simulink model "Frequency_Shift_Keying"  (R2023b)
settings: Solver=VariableStepAuto  StartTime=0.0  StopTime=10.0  RelTol=1e-3
settings Model: Creator=online  LastModifiedBy=online

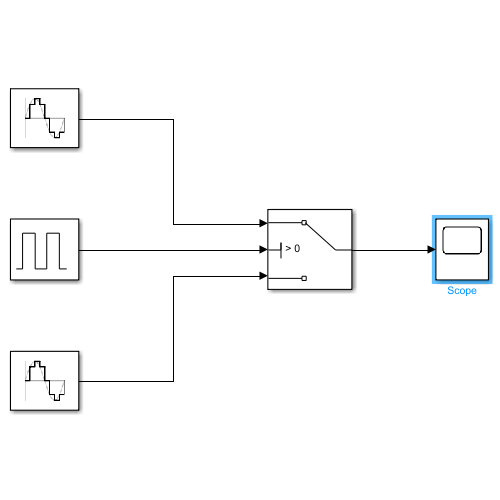
[thumbnail: Simulink's stored preview of the top-level diagram]
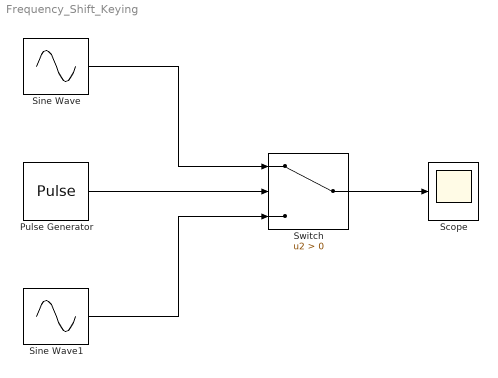
== system Frequency_Shift_Keying ==
  Pulse Generator : DiscretePulseGenerator  PulseType=Time based  Period=1  PulseWidth=50
  Scope : Scope
  Sine Wave : Sin  Frequency=100  SampleTime=0.001
  Sine Wave1 : Sin  Frequency=25  SampleTime=0.001
  Switch : Switch  Criteria=u2 > Threshold  SaturateOnIntegerOverflow=off  InputSameDT=off
  wires:
  Pulse Generator/1 -> Switch/2
  Sine Wave/1 -> Switch/1
  Sine Wave1/1 -> Switch/3
  Switch/1 -> Scope/1
